simulink model "QPSK_ad9361_Solution"  (R2019a)
settings: Solver=ode23  StartTime=0.0  StopTime=inf  RelTol=1e-3  EnableMultiTasking=on
PreLoadFcn:
  | addpath('./filterwizard');
  | ad9361_preload(bdroot,'rx');
  | sdrqpsktx = qpsktx_init;
  | sdrqpskrx = qpskrx_init;
InitFcn:
  | sdrqpsktx = qpsktx_init;
  | sdrqpskrx = qpskrx_init;
undefined symbols (not defined in the file or in its folder): D, dBc, dBval, DCLeak_Matrix, dfilt, doppler, errordlg, Frame, fuzz_val, GainImb_Matrix, gcbh, IP2_Matrix, IP3_Matrix, magnitude, rcfiltgaincompat
libraries: simrfV2elements x23, dspmlti4 x10, simrfV2util1 x9, simulink x9, dsparch4 x8, fl_lib x7, dspmathops x5, dspobslib x4, simrfV2sources1 x3, simrfV2junction1 x3, commdigbbndpm3 x3, dspstat3 x3
(part 2 of 3)

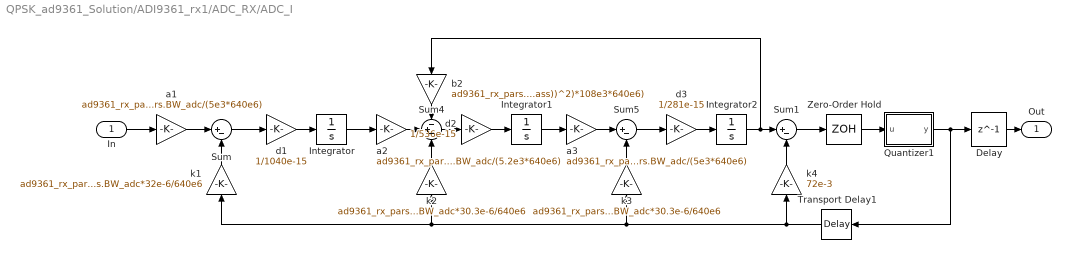
== system QPSK_ad9361_Solution/ADI9361_rx1/ADC_RX/ADC_I ==
  In : Inport
  Delay : Delay  DelayLength=1
  Integrator : Integrator  LimitOutput=on  UpperSaturationLimit=0.9  LowerSaturationLimit=-0.9
  Integrator1 : Integrator  LimitOutput=on  UpperSaturationLimit=0.9  LowerSaturationLimit=-0.9
  Integrator2 : Integrator  LimitOutput=on  UpperSaturationLimit=0.9  LowerSaturationLimit=-0.9
  Quantizer1 : Subsystem
  Sum : Sum  Inputs=|+-
  Sum1 : Sum  Inputs=|+-
  Sum4 : Sum  Inputs=-+-
  Sum5 : Sum  Inputs=|+-
  Transport Delay1 : TransportDelay  DelayTime=ad9361_rx_pars.Tadc/2
  Zero-Order Hold : ZeroOrderHold  SampleTime=ad9361_rx_pars.Tadc
  a1 : Gain  Gain=ad9361_rx_pars.BW_adc/(5e3*640e6)
  a2 : Gain  Gain=ad9361_rx_pars.BW_adc/(5.2e3*640e6)
  a3 : Gain  Gain=ad9361_rx_pars.BW_adc/(5e3*640e6)
  b2 : Gain  Gain=ad9361_rx_pars.BW_adc*1024/(4*((ad9361_rx_pars.BW_adc/(2*ad9361_rx_pars.Fpass))^2)*108e3*640e6)
  d1 : Gain  Gain=1/1040e-15
  d2 : Gain  Gain=1/536e-15
  d3 : Gain  Gain=1/281e-15
  k1 : Gain  Gain=ad9361_rx_pars.BW_adc*32e-6/640e6
  k2 : Gain  Gain=ad9361_rx_pars.BW_adc*30.3e-6/640e6
  k3 : Gain  Gain=ad9361_rx_pars.BW_adc*30.3e-6/640e6
  k4 : Gain  Gain=72e-3
  Out : Outport
  wires:
  k1/1 -> Sum/2
  a1/1 -> Sum/1
  Sum5/1 -> d3/1
  Sum4/1 -> d2/1
  d3/1 -> Integrator2/1
  In/1 -> a1/1
  Integrator2/1 -> Sum1/1, b2/1
  d2/1 -> Integrator1/1
  Integrator1/1 -> a3/1
  d1/1 -> Integrator/1
  Integrator/1 -> a2/1
  Sum/1 -> d1/1
  Zero-Order Hold/1 -> Quantizer1/1(u)
  a2/1 -> Sum4/2
  k2/1 -> Sum4/3
  k3/1 -> Sum5/2
  b2/1 -> Sum4/1
  a3/1 -> Sum5/1
  Sum1/1 -> Zero-Order Hold/1
  k4/1 -> Sum1/2
  Quantizer1/1(y) -> Transport Delay1/1, Delay/1
  Transport Delay1/1 -> k4/1, k1/1, k2/1, k3/1
  Delay/1 -> Out/1

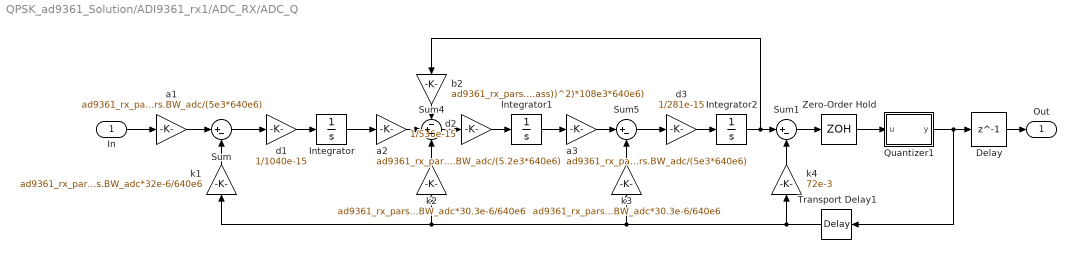
== system QPSK_ad9361_Solution/ADI9361_rx1/ADC_RX/ADC_Q ==
  In : Inport
  Delay : Delay  DelayLength=1
  Integrator : Integrator  LimitOutput=on  UpperSaturationLimit=0.9  LowerSaturationLimit=-0.9
  Integrator1 : Integrator  LimitOutput=on  UpperSaturationLimit=0.9  LowerSaturationLimit=-0.9
  Integrator2 : Integrator  LimitOutput=on  UpperSaturationLimit=0.9  LowerSaturationLimit=-0.9
  Quantizer1 : Subsystem
  Sum : Sum  Inputs=|+-
  Sum1 : Sum  Inputs=|+-
  Sum4 : Sum  Inputs=-+-
  Sum5 : Sum  Inputs=|+-
  Transport Delay1 : TransportDelay  DelayTime=ad9361_rx_pars.Tadc/2
  Zero-Order Hold : ZeroOrderHold  SampleTime=ad9361_rx_pars.Tadc
  a1 : Gain  Gain=ad9361_rx_pars.BW_adc/(5e3*640e6)
  a2 : Gain  Gain=ad9361_rx_pars.BW_adc/(5.2e3*640e6)
  a3 : Gain  Gain=ad9361_rx_pars.BW_adc/(5e3*640e6)
  b2 : Gain  Gain=ad9361_rx_pars.BW_adc*1024/(4*((ad9361_rx_pars.BW_adc/(2*ad9361_rx_pars.Fpass))^2)*108e3*640e6)
  d1 : Gain  Gain=1/1040e-15
  d2 : Gain  Gain=1/536e-15
  d3 : Gain  Gain=1/281e-15
  k1 : Gain  Gain=ad9361_rx_pars.BW_adc*32e-6/640e6
  k2 : Gain  Gain=ad9361_rx_pars.BW_adc*30.3e-6/640e6
  k3 : Gain  Gain=ad9361_rx_pars.BW_adc*30.3e-6/640e6
  k4 : Gain  Gain=72e-3
  Out : Outport
  wires:
  Delay/1 -> Out/1
  Transport Delay1/1 -> k3/1, k2/1, k1/1, k4/1
  Quantizer1/1(y) -> Transport Delay1/1, Delay/1
  k4/1 -> Sum1/2
  Sum1/1 -> Zero-Order Hold/1
  a3/1 -> Sum5/1
  b2/1 -> Sum4/1
  k3/1 -> Sum5/2
  k2/1 -> Sum4/3
  a2/1 -> Sum4/2
  Zero-Order Hold/1 -> Quantizer1/1(u)
  Sum/1 -> d1/1
  Integrator/1 -> a2/1
  d1/1 -> Integrator/1
  Integrator1/1 -> a3/1
  d2/1 -> Integrator1/1
  Integrator2/1 -> b2/1, Sum1/1
  In/1 -> a1/1
  d3/1 -> Integrator2/1
  Sum4/1 -> d2/1
  Sum5/1 -> d3/1
  a1/1 -> Sum/1
  k1/1 -> Sum/2

== system QPSK_ad9361_Solution/ADI9361_rx1/Average Power Meter/Peak Detector ==
  In : Inport
  HTh_i : Constant  Value=Hthreshold_i  SampleTime=ad9361_rx_pars.Tpow*Ncycles
  HTh_o : Constant  Value=Hthreshold_o  SampleTime=ad9361_rx_pars.Tpow*Ncycles
  HighThreshold : RelationalOperator  OutDataTypeStr=boolean  RndMeth=Nearest
  HighThreshold1 : RelationalOperator  Operator=<=  OutDataTypeStr=boolean  RndMeth=Nearest
  LTh_i : Constant  Value=Lthreshold_i  SampleTime=ad9361_rx_pars.Tpow*Ncycles
  LTh_o : Constant  Value=Lthreshold_o  SampleTime=ad9361_rx_pars.Tpow*Ncycles
  LowThreshold : RelationalOperator  OutDataTypeStr=boolean  RndMeth=Nearest
  LowThreshold1 : RelationalOperator  Operator=<=  OutDataTypeStr=boolean  RndMeth=Nearest
  Outer_HTh : Outport
  Inner_HTh : Outport  Port=2
  Inner_LTh : Outport  Port=3
  Outer_LTh : Outport  Port=4
  wires:
  LowThreshold/1 -> Inner_HTh/1
  HighThreshold/1 -> Outer_HTh/1
  HTh_i/1 -> LowThreshold/2
  HTh_o/1 -> HighThreshold/2
  LTh_o/1 -> LowThreshold1/2
  In/1 -> HighThreshold/1, LowThreshold1/1, HighThreshold1/1, LowThreshold/1
  LTh_i/1 -> HighThreshold1/2
  HighThreshold1/1 -> Inner_LTh/1
  LowThreshold1/1 -> Outer_LTh/1

== system QPSK_ad9361_Solution/ADI9361_rx1/Average Power Meter/RMS ==
  In : Inport
  CountNCycles : Buffer  N=Ncycles
  Frame Conversion : FrameConversion  OutFrame=Sample-based
  Gain2 : Gain  Gain=1/Ncycles
  Root : Sqrt  SaturateOnIntegerOverflow=on
  Squared : Math  Operator=magnitude^2  SaturateOnIntegerOverflow=on
  Sum : Sum  Inputs=+
  Out : Outport
  wires:
  Sum/1 -> Gain2/1
  Frame Conversion/1 -> Out/1
  CountNCycles/1 -> Squared/1
  Squared/1 -> Sum/1
  Root/1 -> Frame Conversion/1
  Gain2/1 -> Root/1
  In/1 -> CountNCycles/1

== system QPSK_ad9361_Solution/ADI9361_rx1/Average Power Meter/dB Conversion ==
  in : Inport
  Constant : Constant  Value=fuzz_val  OutDataTypeStr=Inherit: Inherit via back propagation  SampleTime=ad9361_rx_pars.Tpow*Ncycles
  Constant1 : Constant  Value=dBval  OutDataTypeStr=Inherit: Inherit via back propagation  SampleTime=ad9361_rx_pars.Tpow*Ncycles
  Err if non-flt : dspsigattribs/Check Signal Attributes  SigAttribCheckMethod=Does not match attributes exactly  Complexity=Ignore  Frame=Ignore  DimsCheckMethod=Ignore  Dimensions=1-D  DatatypeCheckMethod=Is...  DatatypeGeneral=Floating-point  DtypeFloatSpecific=Any floating-point  DtypeFixedSpecific=Any fixed-point  DtypeIntSpecific=Any integer  SampleMode=Ignore
      settings: SourceProductName=DSP System Toolbox  SourceProductBaseCode=DS
  Error if Cplx : dspsigattribs/Check Signal Attributes  SigAttribCheckMethod=Matches attributes exactly  Complexity=Complex  Frame=Ignore  DimsCheckMethod=Ignore  Dimensions=1-D  DatatypeCheckMethod=Ignore  DatatypeGeneral=Boolean  DtypeFloatSpecific=Any floating-point  DtypeFixedSpecific=Any fixed-point  DtypeIntSpecific=Any integer  SampleMode=Ignore
      settings: SourceProductName=DSP System Toolbox  SourceProductBaseCode=DS
  Gain : Gain  Gain=10  SaturateOnIntegerOverflow=on  OutDataTypeStr=Inherit: Same as input  ParamDataTypeStr=Inherit: Same as input
  Magsq : Math  Operator=magnitude^2  SaturateOnIntegerOverflow=on
  Scale by R : Gain  Gain=1./R  SaturateOnIntegerOverflow=on  OutDataTypeStr=Inherit: Same as input  ParamDataTypeStr=Inherit: Same as input
  Sum1 : Sum  SaturateOnIntegerOverflow=on  InputSameDT=on  OutDataTypeStr=Inherit: Same as first input
  Sum2 : Sum  SaturateOnIntegerOverflow=on  InputSameDT=on  OutDataTypeStr=Inherit: Same as first input
  log10 : Math  Operator=log10  SaturateOnIntegerOverflow=on
  out : Outport  InitialOutput=0
  wires:
  log10/1 -> Gain/1
  Magsq/1 -> Scale by R/1
  Scale by R/1 -> log10/1
  Err if non-flt/1 -> Error if Cplx/1
  in/1 -> Err if non-flt/1
  Error if Cplx/1 -> Sum1/1
  Sum1/1 -> Magsq/1
  Constant/1 -> Sum1/2
  Gain/1 -> Sum2/1
  Sum2/1 -> out/1
  Constant1/1 -> Sum2/2

== system QPSK_ad9361_Solution/ADI9361_rx1/DDC_Filters_RX/Hm1 ==
  note: 1) Only subsystems can be added as variant choices at this level
      | 2) Blocks cannot be connected at this level as connectivity is
      | automatically determined at simulation, based on the active variant
  In : Inport
  Hm1 : Subsystem  VariantControl=(default)
  NoFilter : Subsystem  VariantControl=ad9361_rx_hm1Filt==0
  Out : Outport

== system QPSK_ad9361_Solution/ADI9361_rx1/DDC_Filters_RX/Hm2 ==
  note: 1) Only subsystems can be added as variant choices at this level
      | 2) Blocks cannot be connected at this level as connectivity is
      | automatically determined at simulation, based on the active variant
  In : Inport
  Hm2 : Subsystem  VariantControl=(default)
  NoFilter : Subsystem  VariantControl=ad9361_rx_hm2Filt==0
  Out : Outport

== system QPSK_ad9361_Solution/ADI9361_rx1/DDC_Filters_RX/Hm3 ==
  note: 1) Only subsystems can be added as variant choices at this level
      | 2) Blocks cannot be connected at this level as connectivity is
      | automatically determined at simulation, based on the active variant
  In : Inport
  Hm3 : Subsystem  VariantControl=(default)
  NoFilter : Subsystem  VariantControl=ad9361_rx_hm3Filt==0
  Out : Outport

== system QPSK_ad9361_Solution/ADI9361_rx1/DDC_Filters_RX/Hm4 ==
  note: 1) Only subsystems can be added as variant choices at this level
      | 2) Blocks cannot be connected at this level as connectivity is
      | automatically determined at simulation, based on the active variant
  In1 : Inport
  Hm4 : Subsystem  VariantControl=(default)
  NoFilter : Subsystem  VariantControl=ad9361_rx_hm4Filt==0
  Out1 : Outport

== system QPSK_ad9361_Solution/ADI9361_rx1/LPF_RX/dB2lin ==
  In : Inport
  1/20 : Gain  Gain=1/20
  exp : Math  Operator=10^u  SaturateOnIntegerOverflow=on
  Out : Outport
  wires:
  exp/1 -> Out/1
  In/1 -> 1/20/1
  1/20/1 -> exp/1

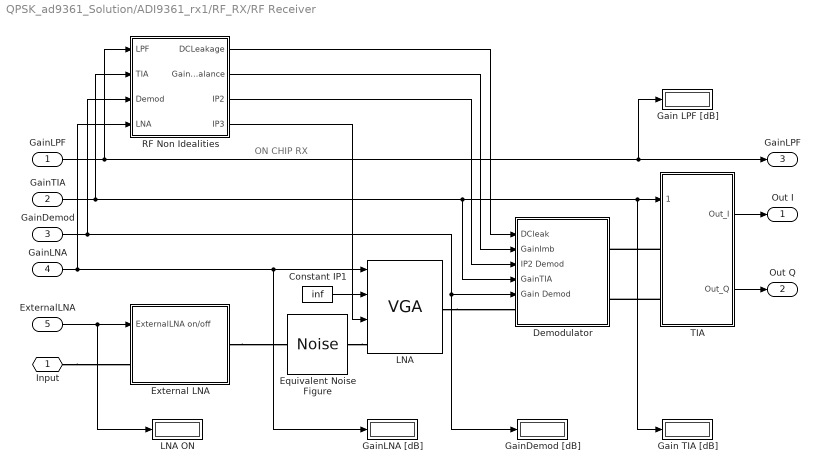
== system QPSK_ad9361_Solution/ADI9361_rx1/RF_RX/RF Receiver ==
  note: ON CHIP RX
  GainLPF : Inport
  GainTIA : Inport  Port=2
  GainDemod : Inport  Port=3
  GainLNA : Inport  Port=4
  ExternalLNA : Inport  Port=5
  Constant IP1 : Constant  Value=inf
  Demodulator : Subsystem
  Equivalent Noise Figure : simrfV2sources1/Noise  SimulinkInputSignalType=Ideal voltage  NoiseType=White  NoisePSD=4*1.381e-23*290*50*10^(NF/10)  CarrierFreq=fc_RF Hz  InternalGrounding=off
      settings: SourceProductName=RF Blockset  SourceProductBaseCode=RB
  External LNA : Subsystem
  Gain LPF [dB] : Display
  Gain TIA [dB] : Display
  GainDemod [dB] : Display
  GainLNA [dB] : Display
  LNA : simrfV2elements/VGA  classname=vga  Zin=Rin  Zout=50  IO=Input  InternalGrounding=on
      settings: SourceProductName=RF Blockset  SourceProductBaseCode=RB
  LNA ON : Display
  RF Non Idealities : Subsystem
  TIA : Subsystem
  Input : PMIOPort  Side=Left
  Out I : Outport
  Out Q : Outport  Port=2
  "GainLPF " : Outport  Port=3
  wires:
  GainTIA/1 -> RF Non Idealities/2(TIA), Gain TIA [dB]/1, TIA/1(Gain TIA), Demodulator/4(GainTIA)
  TIA/1(Out_I) -> Out I/1
  TIA/2(Out_Q) -> Out Q/1
  GainDemod/1 -> RF Non Idealities/3(Demod), Demodulator/5(Gain Demod), GainDemod [dB]/1
  GainLNA/1 -> LNA/1, GainLNA [dB]/1, RF Non Idealities/4(LNA)
  GainLPF/1 -> "GainLPF "/1, Gain LPF [dB]/1, RF Non Idealities/1(LPF)
  RF Non Idealities/1(DCLeakage) -> Demodulator/1(DCleak)
  RF Non Idealities/3(IP2) -> Demodulator/3(IP2 Demod)
  RF Non Idealities/4(IP3) -> LNA/3
  Constant IP1/1 -> LNA/2
  ExternalLNA/1 -> LNA ON/1, External LNA/1(ExternalLNA on/off)
  RF Non Idealities/2(GainImbalance) -> Demodulator/2(GainImb)
  connections:
  LNA/RConn1 -- Demodulator/LConn1
  TIA/LConn1 -- Demodulator/RConn1
  TIA/LConn2 -- Demodulator/RConn2
  Equivalent Noise Figure/LConn1 -- LNA/LConn1
  Input/RConn1 -- External LNA/LConn1
  External LNA/RConn1 -- Equivalent Noise Figure/RConn1

== system QPSK_ad9361_Solution/ADI9361_rx1/Subsystem6/Subsystem1 ==
  Data Type Conversion : DataTypeConversion  OutDataTypeStr=boolean
  Pulse Generator2 : DiscretePulseGenerator  SampleTime=Trf
  START : Outport
  wires:
  Pulse Generator2/1 -> Data Type Conversion/1
  Data Type Conversion/1 -> START/1

== system QPSK_ad9361_Solution/ADI9361_rx1/Subsystem6/Subsystem2 ==
  s : Inport
  w : Inport  Port=2
  Data Type Conversion : DataTypeConversion  OutDataTypeStr=boolean
  Subtract1 : Sum  Inputs=-+  OutDataTypeStr=int8
  os : Outport
  ow : Outport  Port=2
  wires:
  s/1 -> Subtract1/2, os/1
  Data Type Conversion/1 -> ow/1
  Subtract1/1 -> Data Type Conversion/1
  w/1 -> Subtract1/1

== system QPSK_ad9361_Solution/ADI9361_rx1/Subsystem6/Subsystem3 ==
  w : Inport
  s : Inport  Port=2
  Data Type Conversion : DataTypeConversion  OutDataTypeStr=boolean
  Subtract1 : Sum  Inputs=-+  OutDataTypeStr=int8
  ow : Outport
  os : Outport  Port=2
  wires:
  w/1 -> Subtract1/1
  Subtract1/1 -> Data Type Conversion/1
  Data Type Conversion/1 -> ow/1
  s/1 -> Subtract1/2, os/1

== system QPSK_ad9361_Solution/ADI9361_rx1/Subsystem6/Wblk4 ==
  Win : Inport
  Sin : Inport  Port=2
  Combinatorial Logic : CombinatorialLogic  TruthTable=[0; 0; 1; 0]
  Mux : Mux  Inputs=2
  Wout : Outport
  wires:
  Mux/1 -> Combinatorial Logic/1
  Combinatorial Logic/1 -> Wout/1  "wout"
  Win/1 -> Mux/1
  Sin/1 -> Mux/2

== system QPSK_ad9361_Solution/ADI9361_rx1/Subsystem6/Wblk4a ==
  Win : Inport
  Sin : Inport  Port=2
  Combinatorial Logic : CombinatorialLogic  TruthTable=[0; 0; 1; 0]
  Mux : Mux  Inputs=2
  Wout : Outport
  wires:
  Mux/1 -> Combinatorial Logic/1
  Combinatorial Logic/1 -> Wout/1  "wout"
  Win/1 -> Mux/1
  Sin/1 -> Mux/2

== system QPSK_ad9361_Solution/ADI9361_rx1/Subsystem6/Wblk5 ==
  Win : Inport
  Sin : Inport  Port=2
  Combinatorial Logic : CombinatorialLogic  TruthTable=[0; 0; 1; 0]
  Mux : Mux  Inputs=2
  Wout : Outport
  wires:
  Mux/1 -> Combinatorial Logic/1
  Combinatorial Logic/1 -> Wout/1  "wout"
  Win/1 -> Mux/1
  Sin/1 -> Mux/2

== system QPSK_ad9361_Solution/ADI9361_rx1/Subsystem6/Wblk6 ==
  Win : Inport
  Sin : Inport  Port=2
  Combinatorial Logic : CombinatorialLogic  TruthTable=[0; 0; 1; 0]
  Mux : Mux  Inputs=2
  Wout : Outport
  wires:
  Mux/1 -> Combinatorial Logic/1
  Combinatorial Logic/1 -> Wout/1  "wout"
  Win/1 -> Mux/1
  Sin/1 -> Mux/2

== system QPSK_ad9361_Solution/ADI9361_rx1/Subsystem6/Wblk7 ==
  Win : Inport
  Sin : Inport  Port=2
  Combinatorial Logic : CombinatorialLogic  TruthTable=[0; 0; 1; 0]
  Mux : Mux  Inputs=2
  Wout : Outport
  wires:
  Mux/1 -> Combinatorial Logic/1
  Combinatorial Logic/1 -> Wout/1  "wout"
  Win/1 -> Mux/1
  Sin/1 -> Mux/2

== system QPSK_ad9361_Solution/ADI9361_tx1/DUC_Filters_TX/Hm1 ==
  note: 1) Only subsystems can be added as variant choices at this level
      | 2) Blocks cannot be connected at this level as connectivity is
      | automatically determined at simulation, based on the active variant
  In : Inport
  Hm1 : Subsystem  VariantControl=(default)
  NoFilter : Subsystem  VariantControl=ad9361_tx_hm1Filt==0
  Out : Outport

== system QPSK_ad9361_Solution/ADI9361_tx1/DUC_Filters_TX/Hm2 ==
  note: 1) Only subsystems can be added as variant choices at this level
      | 2) Blocks cannot be connected at this level as connectivity is
      | automatically determined at simulation, based on the active variant
  In : Inport
  Hm2 : Subsystem  VariantControl=(default)
  NoFilter : Subsystem  VariantControl=ad9361_tx_hm2Filt==0
  Out : Outport

== system QPSK_ad9361_Solution/ADI9361_tx1/DUC_Filters_TX/Hm3 ==
  note: 1) Only subsystems can be added as variant choices at this level
      | 2) Blocks cannot be connected at this level as connectivity is
      | automatically determined at simulation, based on the active variant
  In : Inport
  Hm3 : Subsystem  VariantControl=(default)
  NoFilter : Subsystem  VariantControl=ad9361_tx_hm3Filt==0
  Out : Outport

== system QPSK_ad9361_Solution/ADI9361_tx1/DUC_Filters_TX/Hm4 ==
  note: 1) Only subsystems can be added as variant choices at this level
      | 2) Blocks cannot be connected at this level as connectivity is
      | automatically determined at simulation, based on the active variant
  In1 : Inport
  Hm4 : Subsystem  VariantControl=(default)
  NoFilter : Subsystem  VariantControl=ad9361_tx_hm4Filt==0
  Out1 : Outport

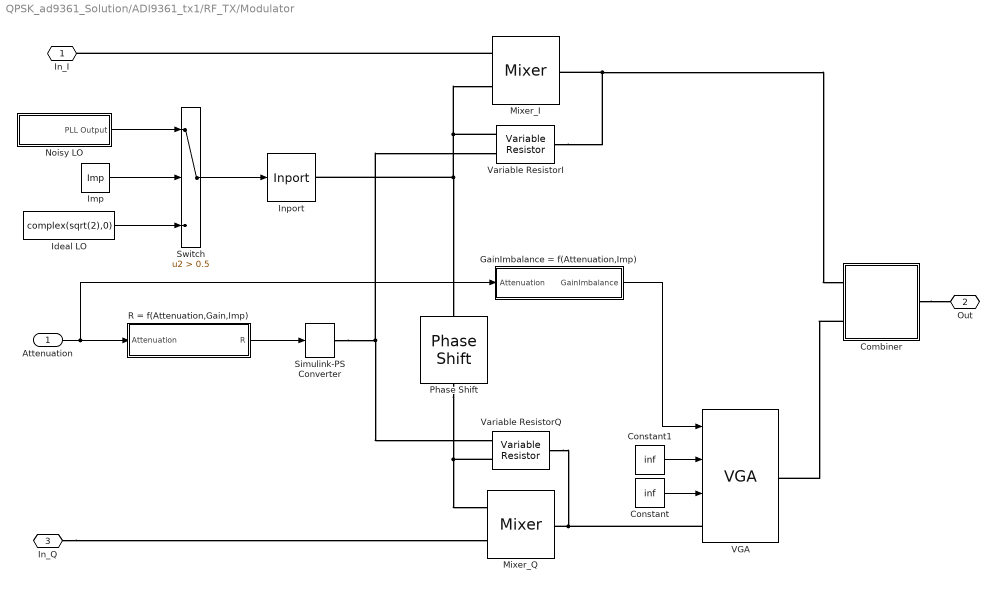
== system QPSK_ad9361_Solution/ADI9361_tx1/RF_TX/Modulator ==
  Attenuation : Inport
  Combiner : Subsystem
  Constant : Constant  Value=inf
  Constant1 : Constant  Value=inf
  GainImbalance = f(Attenuation,Imp) : Subsystem
  Ideal LO : Constant  Value=complex(sqrt(2),0)  SampleTime=Tstep
  Imp : Constant  Value=Imp  SampleTime=Tstep
  Inport : simrfV2util1/Inport  SimulinkInputSignalType=Ideal voltage  CarrierFreq=RF Hz  ZS=0  InternalGrounding=on
      settings: SourceProductName=RF Blockset  SourceProductBaseCode=RB
  Mixer_I : simrfV2elements/Mixer  classname=mixer  Source_linear_gain=Available power gain  linear_gain=0 dB  Zin=50  Zout=50  ZLO=inf  Source_Poly=Even and odd order  Poly_Coeffs=[0 1]  IPType=Output  IP2=Inf dBm  IP3=Inf dBm  P1dB=Inf dBm  Psat=Inf dBm  Gcomp=Inf dBm  NF=0  InternalGrounding=on
      settings: SourceProductName=RF Blockset  SourceProductBaseCode=RB
  Mixer_Q : simrfV2elements/Mixer  classname=mixer  Source_linear_gain=Available power gain  linear_gain=0 dB  Zin=50  Zout=50  ZLO=inf  Source_Poly=Even and odd order  Poly_Coeffs=[0 1]  IPType=Output  IP2=Inf dBm  IP3=Inf dBm  P1dB=Inf dBm  Psat=Inf dBm  Gcomp=Inf dBm  NF=0  InternalGrounding=on
      settings: SourceProductName=RF Blockset  SourceProductBaseCode=RB
  Noisy LO : Subsystem  mask{Level_dB=PN-6, Freq=freqPN, Fs=1/Tstep, Npts=1024*16, seed=951357}
      mask prompts: Level_dB "Noise Level Vector in dBc/Hz"; Freq "Frequency Vector in Hz"; Fs "Sampling Rate in Hz"; Npts "FIR Filter Kernel Length"; seed "Noise Gen Seed"
  Phase Shift : simrfV2elements/Phase Shift  PhaseShift=90 deg  InternalGrounding=on
      settings: SourceProductName=RF Blockset  SourceProductBaseCode=RB
  R = f(Attenuation,Gain,Imp) : Subsystem
  Simulink-PS Converter : nesl_utility/Simulink-PS Converter  PhysicalDomain=network_engine_domain  SubClassName=ps_input  LeftPortType=input  RightPortType=output  PseudoPeriodic=off  Frequencies=[]  NoiseDistribution=none  NoiseParameters=[]  Unit=1  AffineConversion=off  InputFiltering=off  SimscapeFilterOrder=1  InputFilterTimeConstant=0.001  UdotUserProvided=1
  Switch : Switch  Criteria=u2 > Threshold  Threshold=0.5
  VGA : simrfV2elements/VGA  classname=vga  Zin=50  Zout=50  IO=Input  InternalGrounding=on
      settings: SourceProductName=RF Blockset  SourceProductBaseCode=RB
  Variable ResistorI : fl_lib/Electrical/Electrical Elements/Variable Resistor  Rmin=0 Ohm  i_specify=off  i_priority=None  i=0 A  v_specify=off  v_priority=None  v=0 V
  Variable ResistorQ : fl_lib/Electrical/Electrical Elements/Variable Resistor  Rmin=0 Ohm  i_specify=off  i_priority=None  i=0 A  v_specify=off  v_priority=None  v=0 V
  In_I : PMIOPort  Side=Left
  Out : PMIOPort  Port=2  Side=Right
  In_Q : PMIOPort  Port=3  Side=Left
  wires:
  R = f(Attenuation,Gain,Imp)/1(R) -> Simulink-PS Converter/1
  Attenuation/1 -> R = f(Attenuation,Gain,Imp)/1(Attenuation), GainImbalance = f(Attenuation,Imp)/1(Attenuation)
  Switch/1 -> Inport/1
  Imp/1 -> Switch/2
  Noisy LO/1(PLL Output) -> Switch/1
  Ideal LO/1 -> Switch/3
  GainImbalance = f(Attenuation,Imp)/1(GainImbalance) -> VGA/1
  Constant1/1 -> VGA/2
  Constant/1 -> VGA/3
  connections:
  Phase Shift/RConn1 -- Variable ResistorQ/LConn2 -- Mixer_Q/LConn2
  Mixer_I/LConn1 -- In_I/RConn1
  Inport/RConn1 -- Phase Shift/LConn1 -- Variable ResistorI/LConn2 -- Mixer_I/LConn2
  In_Q/RConn1 -- Mixer_Q/LConn1
  Simulink-PS Converter/RConn1 -- Variable ResistorQ/LConn1 -- Variable ResistorI/LConn1
  Variable ResistorQ/RConn1 -- VGA/LConn1 -- Mixer_Q/RConn1
  Variable ResistorI/RConn1 -- Mixer_I/RConn1 -- Combiner/LConn1
  Combiner/RConn1 -- Out/RConn1
  Combiner/LConn2 -- VGA/RConn1

== system QPSK_ad9361_Solution/ADI9361_tx1/RF_TX/PA ==
  " Attenuation" : Inport
  Constant : Constant  Value=Gain
  Constant1 : Constant  Value=inf
  Equivalent Noise Figure : simrfV2sources1/Noise  SimulinkInputSignalType=Ideal voltage  NoiseType=White  NoisePSD=4*1.381e-23*290*50*10^(NF/10)  CarrierFreq=fc_RF Hz  InternalGrounding=off
      settings: SourceProductName=RF Blockset  SourceProductBaseCode=RB
  OIP3 = f(Attenuation,OIP3v,Imp) : Subsystem
  VGA : simrfV2elements/VGA  classname=vga  Zin=50  Zout=50  IO=Output  InternalGrounding=on
      settings: SourceProductName=RF Blockset  SourceProductBaseCode=RB
  In : PMIOPort  Side=Left
  Out : PMIOPort  Port=2  Side=Right
  wires:
  Constant/1 -> VGA/1
  " Attenuation"/1 -> OIP3 = f(Attenuation,OIP3v,Imp)/1(Attenuation)
  OIP3 = f(Attenuation,OIP3v,Imp)/1(OIP3) -> VGA/3
  Constant1/1 -> VGA/2
  connections:
  In/RConn1 -- VGA/LConn1
  Equivalent Noise Figure/RConn1 -- VGA/RConn1
  Equivalent Noise Figure/LConn1 -- Out/RConn1

== system QPSK_ad9361_Solution/QPSK Receiver/Coarse Frequency Compensation1/Find Frequency Offset ==
  note: Algorithm:
      | 1.  Introduce nonlinearity to create tone at M*Foffset, where M is modulation order
      | 2.  Find index of tone within FFT vector
      | 3.  Compute frequency offset
  In : Inport
  Alphabet size : Constant  Value=M  OutDataTypeStr=Inherit: Inherit via back propagation
  Complex Power : commblksprivate/Complex Power
      settings: SourceProductName=Communications Toolbox  SourceProductBaseCode=CM
  Find Frequency Offset : MATLAB Function  TreatAsAtomicUnit=on
  Periodogram : dspspect3/Periodogram  measurement=Power spectral density  wintype=Hamming  Rs=50  beta=5  winsamp=Symmetric  FFTImplementation=Auto  inheritFFT=off  fftsize=2048  navg=16  inheritTs=on  Ts=1
      settings: SourceProductName=DSP System Toolbox  SourceProductBaseCode=DS
  Probe : Probe  ProbeComplexSignal=off
  Frq : Outport
  wires:
  Periodogram/1 -> Find Frequency Offset/3(FFTSig)
  Alphabet size/1 -> Complex Power/2
  In/1 -> Complex Power/1
  Probe/1 -> Find Frequency Offset/1(N)
  Probe/2 -> Find Frequency Offset/2(Tf)
  Find Frequency Offset/1(FreqOffset) -> Frq/1
  Complex Power/1 -> Probe/1, Periodogram/1

== system QPSK_ad9361_Solution/QPSK Receiver/Data Decoding1/Barker Code Symbol Generation  ==
  note: Regenerate a QPSK-modulated unipolar Barker code sequence
      | to be compared with the received data
  Constant Barker Code : Constant  Value=|  VectorParams1D=off
      | [+1 +1 +1 +1 +1 -1 -1 +1 +1 -1 +1 -1 +1
      | ].' > 0
      settings: SamplingMode=Frame based
  Data Type Conversion : DataTypeConversion  OutDataTypeStr=double
  QPSK Modulator Baseband : commdigbbndpm3/QPSK Modulator Baseband  InType=Bit  Enc=Gray  Ph=pi/4  outDtype=double  outWordLen=16  outUDDataType=sfix(16)  outFracLenMode=Best precision  outFracLen=15  outDataTypeStr=double  outLastDataTypeStr=double
      settings: SourceProductName=Communications Toolbox
  Repeat : dspsigops/Repeat  N=2  InputProcessing=Columns as channels (frame based)  RateOptions=Enforce single-rate processing  ic=0  mode=Unused parameter value
      settings: SourceProductName=DSP System Toolbox
  Out : Outport
  wires:
  Constant Barker Code/1 -> Data Type Conversion/1
  Repeat/1 -> QPSK Modulator Baseband/1
  QPSK Modulator Baseband/1 -> Out/1
  Data Type Conversion/1 -> Repeat/1

== system QPSK_ad9361_Solution/QPSK Receiver/Data Decoding1/Compute Delay ==
  note: Correlation with the modulated symbols
  Barker Reference : Inport
  Data : Inport  Port=2
  Abs : Abs
  Constant1 : Constant  VectorParams1D=off  OutDataTypeStr=Inherit: Inherit via back propagation  FramePeriod=2
  Correlation : dspstat3/Correlation  domain=Time  roundingMode=Floor  overflowMode=off  accumDataTypeStr=Inherit: Same as product output  accumLastDataTypeStr=Inherit: Same as product output  outputDataTypeStr=Inherit: Same as accumulator  outputMin=[]  outputMax=[]  outputLastDataTypeStr=Inherit: Same as accumulator
      settings: SourceProductName=DSP System Toolbox  SourceProductBaseCode=DS
  Math Function : Math  Operator=mod  SaturateOnIntegerOverflow=on
  Maximum : dspstat3/Maximum  operation=maximum  fcn=Index  indexBase=One  operateOver=Each column  Dimension=1  InputProcessing=Columns as channels (frame based)  reset=None  roiEnable=off  roiType=Rectangles  roiPortion=Entire ROI  roiOutput=Individual statistics for each ROI  roiFlag=off  roundingMode=Floor  overflowMode=off  accumDataTypeStr=Inherit: Same as product output  accumLastDataTypeStr=Inherit: Same as product output
  Probe : Probe  ProbeSampleTime=off  ProbeComplexSignal=off
  Sum : Sum  Inputs=|-+  SaturateOnIntegerOverflow=on  InputSameDT=on  OutDataTypeStr=Inherit: Same as first input
  Sum1 : Sum  Inputs=|+-  SaturateOnIntegerOverflow=on  InputSameDT=on  OutDataTypeStr=Inherit: Same as first input
  Delay : Outport
  wires:
  Abs/1 -> Maximum/1
  Constant1/1 -> Sum1/2
  Sum1/1 -> Math Function/2
  Math Function/1 -> Delay/1
  Sum/1 -> Math Function/1
  Probe/1 -> Sum1/1, Sum/2
  Correlation/1 -> Abs/1
  Maximum/1 -> Sum/1
  Barker Reference/1 -> Correlation/1
  Data/1 -> Correlation/2, Probe/1

== system QPSK_ad9361_Solution/QPSK Receiver/Data Decoding1/Descrambling ==
  In : Inport
  Descrambler : commsequence2/Descrambler  M=2  poly=[1 1 1 0 1]  iniStaSource=Dialog Parameter  ini_sta=[0 0 0 0]  resetViaPort=off
      settings: SourceProductName=Communications Toolbox  SourceProductBaseCode=CM
  Selector : Selector  IndexOptions=Index vector (dialog)  Indices=[sdrqpskrx.BarkerLength*log2(sdrqpskrx.M)+1:sdrqpskrx.FrameSize*log2(sdrqpskrx.M)]  OutputSizes=1
  Selector1 : Selector  IndexOptions=Index vector (dialog)  Indices=[1:sdrqpskrx.MsgLength]  OutputSizes=1
  Out : Outport
  wires:
  Descrambler/1 -> Selector1/1
  Selector1/1 -> Out/1
  In/1 -> Selector/1
  Selector/1 -> Descrambler/1

== system QPSK_ad9361_Solution/QPSK Receiver/Data Decoding1/Phase Ambiguity Correction & Demodulation ==
  note: Phase Ambiguity Resolution
      | and Demodulation
  Phase : Inport
  Data : Inport  Port=2
  Complex Phase Shift : commutil2/Complex Phase Shift
      settings: SourceProductName=Communications Toolbox  SourceProductBaseCode=CM
  Constellation RX : ConstellationDiagram
  Gain : Gain  Gain=-1
  QPSK Demodulator Baseband : commdigbbndpm3/QPSK Demodulator Baseband  OutType=Bit  DecType=Hard decision  VarSource=Dialog  Variance=1  Dec=Gray  Ph=pi/4  outDtype1=Inherit via internal rule  outDtype2=Inherit via internal rule  derotateFactorWordLen=16  derotateFactorDataTypeStr=Inherit: Same word length as input  derotateFactorLastDataTypeStr=Inherit: Same word length as input
      settings: SourceProductName=Communications Toolbox
  Out : Outport
  wires:
  Phase/1 -> Gain/1
  Data/1 -> Complex Phase Shift/1
  Complex Phase Shift/1 -> Constellation RX/1, QPSK Demodulator Baseband/1
  QPSK Demodulator Baseband/1 -> Out/1
  Gain/1 -> Complex Phase Shift/2

== system QPSK_ad9361_Solution/QPSK Receiver/Data Decoding1/Phase Offset Estimator ==
  note: 1. The original signal is expressed as y(t) = x(t)e^{j\phi}+n(t), t = 1, 2, ..., N
      | 2. y_1(t) = x{*}(t)y(t) = e^{j\phi} + x{*}(t)n(t)
      | The goal is to estimate the value \phi from the observation y_1(t), t = 1, 2, ...N
      | i.e., estimate the value B = e^{j\phi}, and \phi = angle(B)
      | 3. Suppose n(t) yields to a i.i.d. complex AWGN distribution N(0,\sigma^2).
      | Then a non-biased estimator could be
      | B_{est} = 1/N*sum(y_1(1:N)), and \phi_{est} = angle(B_{est})
      | and the variance of B_{est} is \sigma^2/N
  BarkerRef : Inport
  Data : Inport  Port=2
  Complex to Magnitude-Angle : ComplexToMagnitudeAngle  Output=Angle
  Math Function : Math  Operator=conj  SaturateOnIntegerOverflow=on
  Mean : dspstat3/Mean  run=off  reset_popup=None  InputProcessing=Columns as channels (frame based)  directionMode=Each column  dimension=1  roiEnable=off  roiType=Rectangles  roiPortion=Entire ROI  roiOutput=Individual statistics for each ROI  roiFlag=off  outputDataTypeStr=Inherit: Same as accumulator  outputLastDataTypeStr=Inherit: Same as accumulator  outputMin=[]  outputMax=[]  roundingMode=Floor  overflowMode=off
  Phase Offset Detection : MATLAB Function  TreatAsAtomicUnit=on
  Product : Product  RndMeth=Zero
  Selector : Selector  IndexOptions=Index vector (dialog)  Indices=[1:sdrqpskrx.BarkerLength]  OutputSizes=1
  Phase : Outport
  wires:
  Data/1 -> Selector/1
  BarkerRef/1 -> Math Function/1  "x(t)"
  Selector/1 -> Product/2  "y(t)"
  Math Function/1 -> Product/1  "x*(t)"
  Product/1 -> Mean/1  "y_1(t)"
  Mean/1 -> Complex to Magnitude-Angle/1
  Complex to Magnitude-Angle/1 -> Phase Offset Detection/1(In)
  Phase Offset Detection/1(Out) -> Phase/1

== system QPSK_ad9361_Solution/QPSK Receiver/Fine Frequency Compensation1/DDS ==
  note: The digital filter acts as a pure integrator
  In : Inport
  Digital Filter : dspobslib/Digital Filter  TypePopup=IIR (poles & zeros)  IIRFiltStruct=Direct form II transposed  AllPoleFiltStruct=Direct form  FIRFiltStruct=Direct form  CoeffSource=Specify via dialog  NumCoeffs=[0 1]  DenCoeffs=[1 -1]  BiQuadCoeffs=[1 0.3 0.4 1 0.1 0.2]  LatticeCoeffs=[0.2 0.4]  denIgnore=on  FiltPerSampPopup=One filter per frame  IC=0  ICnum=0  ICden=0  roundingMode=Floor  overflowMode=off  ScaleValues=1  scaleValueFracLength=14  stageInFracLength=15  stageOutFracLength=15  FilterSource=Specify via dialog  dfiltObjectName=dfilt.dffir([1 2 1])  InputProcessing=Columns as channels (frame based)
      settings: SourceProductName=DSP System Toolbox  SourceProductBaseCode=DS
  Gain : Gain  Gain=-1*sdrqpskrx.FineFreqCompensateGain
  Phase : Outport
  wires:
  Digital Filter/1 -> Gain/1
  In/1 -> Digital Filter/1
  Gain/1 -> Phase/1

== system QPSK_ad9361_Solution/QPSK Receiver/Fine Frequency Compensation1/Loop Filter ==
  note: Proportional-plus-Integrator Loop Filter,
      | Infinite DC Response to guarantee convergence
  e : Inport
  Digital Filter : dspobslib/Digital Filter  TypePopup=IIR (poles & zeros)  IIRFiltStruct=Direct form II transposed  AllPoleFiltStruct=Direct form  FIRFiltStruct=Direct form  CoeffSource=Specify via dialog  NumCoeffs=[1 0]  DenCoeffs=[1 -1]  BiQuadCoeffs=[1 0.3 0.4 1 0.1 0.2]  LatticeCoeffs=[0.2 0.4]  denIgnore=on  FiltPerSampPopup=One filter per frame  IC=0  ICnum=0  ICden=0  roundingMode=Floor  overflowMode=off  ScaleValues=1  scaleValueFracLength=14  stageInFracLength=15  stageOutFracLength=15  FilterSource=Specify via dialog  dfiltObjectName=dfilt.dffir([1 2 1])  InputProcessing=Columns as channels (frame based)
      settings: SourceProductName=DSP System Toolbox  SourceProductBaseCode=DS
  K1 : Gain  Gain=K1
  K2 : Gain  Gain=K2
  Sum2 : Sum  SaturateOnIntegerOverflow=on  InputSameDT=on  OutDataTypeStr=Inherit: Same as first input
  v : Outport
  wires:
  K2/1 -> Digital Filter/1
  Digital Filter/1 -> Sum2/2
  Sum2/1 -> v/1
  e/1 -> K2/1, K1/1
  K1/1 -> Sum2/1

== system QPSK_ad9361_Solution/QPSK Receiver/Timing Recovery1/Modified Buffer ==
  Data : Inport
  Clk : Inport  Port=2
  Logical Operator : Logic  AllPortsSameDT=off  OutDataTypeStr=boolean
  Modified Buffer : Subsystem
  DataOut : Outport
  DataValid : Outport  Port=2
  wires:
  Data/1 -> Modified Buffer/1(In1)
  Clk/1 -> Modified Buffer/Enable, Logical Operator/2
  Modified Buffer/1(DataOut) -> DataOut/1
  Modified Buffer/2(DataValid) -> Logical Operator/1
  Logical Operator/1 -> DataValid/1

== system QPSK_ad9361_Solution/QPSK Receiver/Timing Recovery1/Timing Recovery PLL ==
  note: Sample-based processing is adopted because
      | 1. Strobe signal is required to generate for EVERY sample for processing and output
      | sampling, delayed strobe signal would affect the accuracy of bit stripping/stuffing
      | 2. The BER performance degrades significantly even with frame size 2 and 4
  note: Baseband implementation of the Symbol Timing Synchronization listed in Chapter 8.4
      | of "Digital Communications- A Discrete-Time Approach" by Michael Rice. See Appendix
      | C.2 of the same book for the details of PLL design.
  note: To determine phase error detector gain K_p, See Equation 8.42 &
      | Figure 8.4.7 of "Digital Communications - A Discrete-Time Approach"
      | by Michael Rice.
  DataIn : Inport
  Integer Delay1 : Delay  DelayLength=1
  Integer Delay2 : Delay  DelayLength=1
  Interpolation Filter : MATLAB Function  TreatAsAtomicUnit=on
  Loop Filter : Subsystem  mask{BnTs=0.01, zeta=1, Kp=sdrqpskrx.TimingRecTEDGain, K0=sdrqpskrx.TimingRecCompensateGain, N=sdrqpskrx.Upsampling/sdrqpskrx.Downsampling}
      mask prompts: BnTs "Loop Bandwidth"; zeta "Loop Damping Factor"; Kp "Phase Detector Gain (Kp)"; K0 "DDS gain (K0)"; N "Number of Samples/symbol (N)"
      mask init:
      | % See C.57 to C.61 in Michael Rice's "Digital Communications 
      | % - A Discrete-Time Approach" for details
      | theta = BnTs/(zeta+0.25/zeta)/N;
      | d = 1 + 2*zeta*theta + theta*theta;
      | K1 = 4*zeta*theta/d;
      | K2 = 4*theta*theta/d;
      | K1 = K1/(Kp*K0);
      | K2 = K2/(Kp*K0);
      mask Display: disp('Loop Filter');
  NCO Control : MATLAB Function
  Timing Error Detector : MATLAB Function  TreatAsAtomicUnit=on
  DataOut : Outport
  ClkOut : Outport  Port=2
  wires:
  DataIn/1 -> Interpolation Filter/1(In)
  NCO Control/2(mu) -> Integer Delay2/1
  Integer Delay1/1 -> ClkOut/1, Timing Error Detector/2(strobe)
  NCO Control/1(Underflow) -> Integer Delay1/1
  Interpolation Filter/1(Out) -> DataOut/1, Timing Error Detector/1(In)
  Loop Filter/1(v) -> NCO Control/1(Delta)
  Timing Error Detector/1(e) -> Loop Filter/1(e)
  Integer Delay2/1 -> Interpolation Filter/2(mu)

== system QPSK_ad9361_Solution/QPSK TX/Bit Generation/Barker Code SS ==
  Constant Barker Code : Constant  Value=|  VectorParams1D=off
      | [+1 +1 +1 +1 +1 -1 -1 +1 +1 -1 +1 -1 +1
      | ].' > 0  % Bipolar to Unipolar Conversion
      settings: SamplingMode=Frame based
  Data Type Conversion : DataTypeConversion  OutDataTypeStr=double
  Out : Outport
  wires:
  Data Type Conversion/1 -> Out/1
  Constant Barker Code/1 -> Data Type Conversion/1

== system QPSK_ad9361_Solution/QPSK TX/Bit Generation/Message Source ==
  Bernoulli Binary Generator : commrandsrc2/Bernoulli Binary Generator  P=0.5  seed=61  Ts=sdrqpsktx.FrameTime/(sdrqpsktx.DataLength-sdrqpsktx.MsgLength)  frameBased=on  sampPerFrame=sdrqpsktx.DataLength-sdrqpsktx.MsgLength  orient=off  outDataType=double
      settings: SourceProductName=Communications Toolbox  SourceProductBaseCode=CM
  Matrix Concatenate : Concatenate  Mode=Multidimensional array
  Message Generator : MATLAB Function  TreatAsAtomicUnit=on
  Out : Outport
  wires:
  Matrix Concatenate/1 -> Out/1
  Bernoulli Binary Generator/1 -> Matrix Concatenate/2
  Message Generator/1(msg) -> Matrix Concatenate/1

== system QPSK_ad9361_Solution/ADI9361_rx1/ADC_RX/ADC_I/Quantizer1 ==
  u : Inport
  Abs : Abs
  Idealized ADC quantizer : simulink_extras/Additional Discrete/Idealized ADC quantizer  NumberOfConverterBits=3  Vmin=0  Vmax=.8  OutputDataType=double  OutputNegativeValues=off
      settings: SourceProductName=Simulink
  Product : Product
  Saturation : Saturate  UpperLimit=0.41
  Sign : Signum
  y : Outport
  wires:
  u/1 -> Sign/1, Abs/1
  Saturation/1 -> Idealized ADC quantizer/1
  Idealized ADC quantizer/1 -> Product/1
  Sign/1 -> Product/2
  Abs/1 -> Saturation/1
  Product/1 -> y/1

== system QPSK_ad9361_Solution/ADI9361_rx1/ADC_RX/ADC_Q/Quantizer1 ==
  u : Inport
  Abs : Abs
  Idealized ADC quantizer : simulink_extras/Additional Discrete/Idealized ADC quantizer  NumberOfConverterBits=3  Vmin=0  Vmax=.8  OutputDataType=double  OutputNegativeValues=off
      settings: SourceProductName=Simulink
  Product : Product
  Saturation : Saturate  UpperLimit=0.41
  Sign : Signum
  y : Outport
  wires:
  u/1 -> Sign/1, Abs/1
  Saturation/1 -> Idealized ADC quantizer/1
  Idealized ADC quantizer/1 -> Product/1
  Sign/1 -> Product/2
  Abs/1 -> Saturation/1
  Product/1 -> y/1

== system QPSK_ad9361_Solution/ADI9361_rx1/DDC_Filters_RX/Hm1/Hm1 ==
  In : Inport
  Hm1 : dspmlti4/FIR Decimation  FilterSource=Filter object  h=fir1(35,0.4)  D=2  filtStruct=Direct form  FilterObject=ad9361_rx_pars.Hm1_rx  framing=Allow multirate processing  inputOffset=0  outputBufInitCond=0  roundingMode=Floor  overflowMode=off  firstCoeffDataTypeStr=Inherit: Same word length as input  firstCoeffMin=[]  firstCoeffMax=[]  firstCoeffLastDataTypeStr=Inherit: Same word length as input  outputDataTypeStr=Inherit: Same as accumulator  outputMin=[]  outputMax=[]  outputLastDataTypeStr=Inherit: Same as accumulator
  Out : Outport
  wires:
  In/1 -> Hm1/1
  Hm1/1 -> Out/1

== system QPSK_ad9361_Solution/ADI9361_rx1/DDC_Filters_RX/Hm1/NoFilter ==
  In : Inport
  Out : Outport
  wires:
  In/1 -> Out/1

== system QPSK_ad9361_Solution/ADI9361_rx1/DDC_Filters_RX/Hm2/Hm2 ==
  In : Inport
  Data Type Conversion3 : DataTypeConversion  OutDataTypeStr=fixdt(1,16,14)  RndMeth=Round
  Hm2 : dspmlti4/FIR Decimation  FilterSource=Filter object  h=fir1(35,0.4)  D=2  filtStruct=Direct form  FilterObject=ad9361_rx_pars.Hm2_rx  framing=Allow multirate processing  inputOffset=0  outputBufInitCond=0  roundingMode=Floor  overflowMode=off  firstCoeffDataTypeStr=Inherit: Same word length as input  firstCoeffMin=[]  firstCoeffMax=[]  firstCoeffLastDataTypeStr=Inherit: Same word length as input  outputDataTypeStr=Inherit: Same as accumulator  outputMin=[]  outputMax=[]  outputLastDataTypeStr=Inherit: Same as accumulator
  Out : Outport
  wires:
  In/1 -> Data Type Conversion3/1
  Hm2/1 -> Out/1
  Data Type Conversion3/1 -> Hm2/1

== system QPSK_ad9361_Solution/ADI9361_rx1/DDC_Filters_RX/Hm2/NoFilter ==
  In : Inport
  Data Type Conversion3 : DataTypeConversion  OutDataTypeStr=fixdt(1,16,14)  RndMeth=Round
  Out : Outport
  wires:
  In/1 -> Data Type Conversion3/1
  Data Type Conversion3/1 -> Out/1

== system QPSK_ad9361_Solution/ADI9361_rx1/DDC_Filters_RX/Hm3/Hm3 ==
  In : Inport
  Mh3 : dspmlti4/FIR Decimation  FilterSource=Filter object  h=fir1(35,0.4)  D=2  filtStruct=Direct form  FilterObject=ad9361_rx_pars.Hm3_rx  framing=Allow multirate processing  inputOffset=0  outputBufInitCond=0  roundingMode=Floor  overflowMode=off  firstCoeffDataTypeStr=Inherit: Same word length as input  firstCoeffMin=[]  firstCoeffMax=[]  firstCoeffLastDataTypeStr=Inherit: Same word length as input  outputDataTypeStr=Inherit: Same as accumulator  outputMin=[]  outputMax=[]  outputLastDataTypeStr=Inherit: Same as accumulator
  Out : Outport
  wires:
  In/1 -> Mh3/1
  Mh3/1 -> Out/1

== system QPSK_ad9361_Solution/ADI9361_rx1/DDC_Filters_RX/Hm3/NoFilter ==
  In : Inport
  Out : Outport
  wires:
  In/1 -> Out/1

== system QPSK_ad9361_Solution/ADI9361_rx1/DDC_Filters_RX/Hm4/Hm4 ==
  In1 : Inport
  Data Type Conversion : DataTypeConversion  OutDataTypeStr=fixdt(1,4,2)  RndMeth=Round
  Hm1 : dspmlti4/FIR Decimation  FilterSource=Filter object  h=fir1(35,0.4)  D=2  filtStruct=Direct form  FilterObject=ad9361_rx_pars.Hm4_rx  framing=Allow multirate processing  inputOffset=0  outputBufInitCond=0  roundingMode=Floor  overflowMode=off  firstCoeffDataTypeStr=Inherit: Same word length as input  firstCoeffMin=[]  firstCoeffMax=[]  firstCoeffLastDataTypeStr=Inherit: Same word length as input  outputDataTypeStr=Inherit: Same as accumulator  outputMin=[]  outputMax=[]  outputLastDataTypeStr=Inherit: Same as accumulator
  Out1 : Outport
  wires:
  In1/1 -> Data Type Conversion/1
  Hm1/1 -> Out1/1
  Data Type Conversion/1 -> Hm1/1

== system QPSK_ad9361_Solution/ADI9361_rx1/DDC_Filters_RX/Hm4/NoFilter ==
  In1 : Inport
  Data Type Conversion : DataTypeConversion  OutDataTypeStr=fixdt(1,4,2)  RndMeth=Round
  Out1 : Outport
  wires:
  In1/1 -> Data Type Conversion/1
  Data Type Conversion/1 -> Out1/1

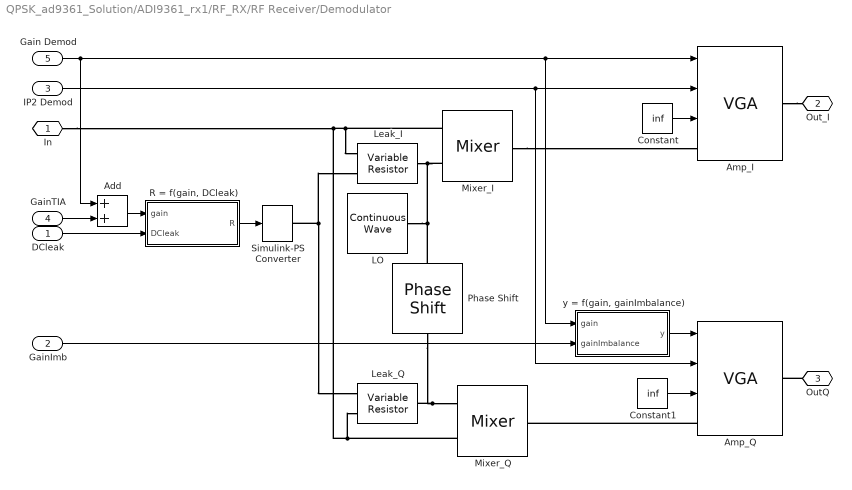
== system QPSK_ad9361_Solution/ADI9361_rx1/RF_RX/RF Receiver/Demodulator ==
  DCleak : Inport
  GainImb : Inport  Port=2
  IP2 Demod : Inport  Port=3
  GainTIA : Inport  Port=4
  Gain Demod : Inport  Port=5
  Add : Sum
  Amp_I : simrfV2elements/VGA  classname=vga  Zin=100  Zout=100  IO=Input  InternalGrounding=on
      settings: SourceProductName=RF Blockset  SourceProductBaseCode=RB
  Amp_Q : simrfV2elements/VGA  classname=vga  Zin=100  Zout=100  IO=Input  InternalGrounding=on
      settings: SourceProductName=RF Blockset  SourceProductBaseCode=RB
  Constant : Constant  Value=inf
  Constant1 : Constant  Value=inf
  LO : simrfV2sources1/Continuous Wave  CWSourceType=Ideal voltage  Z0=0  IVoltage=1/sqrt(2) V  ICurrent=0 A  MagPower=1 W  QVoltage=0 V  QCurrent=0 A  AnglePower=0  CarrierFreq=RF Hz  InternalGrounding=on
      settings: SourceProductName=RF Blockset  SourceProductBaseCode=RB
  Leak_I : fl_lib/Electrical/Electrical Elements/Variable Resistor  Rmin=0 Ohm  i_specify=off  i_priority=High  i=0 A  v_specify=off  v_priority=High  v=0 V
  Leak_Q : fl_lib/Electrical/Electrical Elements/Variable Resistor  Rmin=0 Ohm  i_specify=off  i_priority=High  i=0 A  v_specify=off  v_priority=High  v=0 V
  Mixer_I : simrfV2elements/Mixer  classname=mixer  Source_linear_gain=Available power gain  linear_gain=0 dB  Zin=100  Zout=100  ZLO=inf  Source_Poly=Even and odd order  Poly_Coeffs=[0 1]  IPType=Output  IP2=Inf dBm  IP3=Inf dBm  P1dB=Inf dBm  Psat=Inf dBm  Gcomp=Inf dBm  NF=0  InternalGrounding=on
      settings: SourceProductName=RF Blockset  SourceProductBaseCode=RB
  Mixer_Q : simrfV2elements/Mixer  classname=mixer  Source_linear_gain=Available power gain  linear_gain=0 dB  Zin=100  Zout=100  ZLO=inf  Source_Poly=Even and odd order  Poly_Coeffs=[0 1]  IPType=Output  IP2=Inf dBm  IP3=Inf dBm  P1dB=Inf dBm  Psat=Inf dBm  Gcomp=Inf dBm  NF=0  InternalGrounding=on
      settings: SourceProductName=RF Blockset  SourceProductBaseCode=RB
  Phase Shift : simrfV2elements/Phase Shift  PhaseShift=90 deg  InternalGrounding=on
      settings: SourceProductName=RF Blockset  SourceProductBaseCode=RB
  "R = f(gain, DCleak)" : Subsystem
  Simulink-PS Converter : nesl_utility/Simulink-PS Converter  PhysicalDomain=network_engine_domain  SubClassName=ps_input  LeftPortType=input  RightPortType=output  PseudoPeriodic=off  Frequencies=[]  NoiseDistribution=none  NoiseParameters=[]  Unit=1  AffineConversion=off  InputFiltering=off  SimscapeFilterOrder=1  InputFilterTimeConstant=0.001  UdotUserProvided=1
  "y = f(gain, gainImbalance)" : Subsystem
  In : PMIOPort  Side=Left
  Out_I : PMIOPort  Port=2  Side=Right
  OutQ : PMIOPort  Port=3  Side=Right
  wires:
  Gain Demod/1 -> "y = f(gain, gainImbalance)"/1(gain), Amp_I/1, Add/1
  IP2 Demod/1 -> Amp_Q/2, Amp_I/2
  "R = f(gain, DCleak)"/1(R) -> Simulink-PS Converter/1
  GainTIA/1 -> Add/2
  Add/1 -> "R = f(gain, DCleak)"/1(gain)
  GainImb/1 -> "y = f(gain, gainImbalance)"/2(gainImbalance)
  DCleak/1 -> "R = f(gain, DCleak)"/2(DCleak)
  "y = f(gain, gainImbalance)"/1(y) -> Amp_Q/1
  Constant/1 -> Amp_I/3
  Constant1/1 -> Amp_Q/3
  connections:
  Phase Shift/RConn1 -- Mixer_Q/LConn2 -- Leak_Q/RConn1
  Mixer_I/LConn2 -- Leak_I/RConn1 -- LO/LConn1 -- Phase Shift/LConn1
  Mixer_Q/LConn1 -- Leak_Q/LConn2 -- In/RConn1 -- Leak_I/LConn2 -- Mixer_I/LConn1
  Amp_I/RConn1 -- Out_I/RConn1
  OutQ/RConn1 -- Amp_Q/RConn1
  Mixer_I/RConn1 -- Amp_I/LConn1
  Amp_Q/LConn1 -- Mixer_Q/RConn1
  Simulink-PS Converter/RConn1 -- Leak_Q/LConn1 -- Leak_I/LConn1

== system QPSK_ad9361_Solution/ADI9361_rx1/RF_RX/RF Receiver/External LNA ==
  ExternalLNA on/off : Inport
  Bypass : simrfV2junction1/Switch  classname=switch  Ron=0 Ohm  Roff=inf Ohm  Vthres=0.5 V
      settings: SourceProductName=RF Blockset  SourceProductBaseCode=RB
  Invert Control : Subsystem
  LNA : simrfV2elements/Amplifier  classname=amplifier  DataSource=Data file  File=simrfV2_unitygain.s2p  Paramtype=S-parameters  Sparam=[0 0;1 0]  SparamFreq=1e9 Hz  SparamZ0=50  Residues=0  Poles=0  DF={0 0; 1 0}  Source_linear_gain=Available power gain  linear_gain=10 dB  Zin=50  Zout=50  Source_Poly=Even and odd order  Poly_Coeffs=[0 1]  IPType=Output  IP2=inf dBm  IP3=inf dBm  P1dB=inf dBm  Psat=inf dBm  Gcomp=inf dBm  NF=0  InternalGrounding=on  SourceFreq=Extracted from data source  PlotFreq=[1e9:1e6:3e9] Hz  PlotType=X-Y plane  YParam1=S11  YFormat1=Magnitude (decibels)  YParam2=None  YFormat2=Magnitude (decibels)  YOption=Linear  XOption=Linear  SparamRepresentation=Time domain (rationalfit)  FitTol=-40  FitOpt=Fit individually  AutoImpulseLength=off  ImpulseLength=0 s
      settings: SourceProductName=RF Blockset  SourceProductBaseCode=RB
  LNA on input : simrfV2junction1/Switch  classname=switch  Ron=0 Ohm  Roff=inf Ohm  Vthres=0.5 V
      settings: SourceProductName=RF Blockset  SourceProductBaseCode=RB
  LNA on ouput : simrfV2junction1/Switch  classname=switch  Ron=0 Ohm  Roff=inf Ohm  Vthres=0.5 V
      settings: SourceProductName=RF Blockset  SourceProductBaseCode=RB
  in : PMIOPort  Side=Left
  out : PMIOPort  Port=2  Side=Right
  wires:
  ExternalLNA on/off/1 -> LNA on ouput/1, LNA on input/1, Invert Control/1(In)
  Invert Control/1(Out) -> Bypass/1
  connections:
  Bypass/RConn1 -- out/RConn1 -- LNA on ouput/RConn1
  LNA on input/LConn1 -- Bypass/LConn1 -- in/RConn1
  LNA on input/RConn1 -- LNA/LConn1
  LNA/RConn1 -- LNA on ouput/LConn1

== system QPSK_ad9361_Solution/ADI9361_rx1/RF_RX/RF Receiver/RF Non Idealities ==
  LPF : Inport
  TIA : Inport  Port=2
  Demod : Inport  Port=3
  LNA : Inport  Port=4
  DetectChange : Subsystem
  RF Non Idealities : Subsystem
  DCLeakage : Outport
  GainImbalance : Outport  Port=2
  IP2 : Outport  Port=3
  IP3 : Outport  Port=4
  wires:
  TIA/1 -> RF Non Idealities/3(TIA), DetectChange/3(In3)
  LPF/1 -> RF Non Idealities/4(LPF), DetectChange/4(In4)
  Demod/1 -> RF Non Idealities/2(Demod), DetectChange/2(In2)
  LNA/1 -> RF Non Idealities/1(LNA), DetectChange/1(In1)
  RF Non Idealities/1(DCLeakage) -> DCLeakage/1
  RF Non Idealities/2(GainImbalance) -> GainImbalance/1
  RF Non Idealities/3(IP2) -> IP2/1
  RF Non Idealities/4(IP3) -> IP3/1
  DetectChange/1(Trigger) -> RF Non Idealities/Trigger

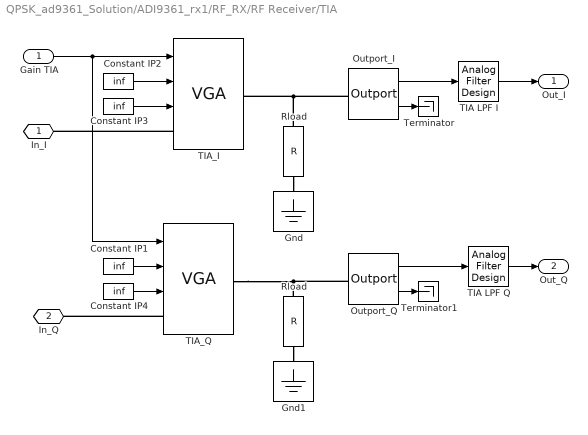
== system QPSK_ad9361_Solution/ADI9361_rx1/RF_RX/RF Receiver/TIA ==
  Gain TIA : Inport
  " Rload" : simrfV2elements/R  classname=resistor  Resistance=100 Ohm  AddNoise=on
      settings: SourceProductName=RF Blockset  SourceProductBaseCode=RB
  Constant IP{1..4} (4 alike) : Constant  Value=inf
  Gnd : fl_lib/Electrical/Electrical Elements/Electrical Reference
  Gnd1 : fl_lib/Electrical/Electrical Elements/Electrical Reference
  Outport_I : simrfV2util1/Outport  SensorType=Ideal voltage  OutputFormat=In-phase and Quadrature Baseband  CarrierFreq=0 Hz  ZL=Inf  InternalGrounding=on  StepSize=-1 s  AutoStep=off
      settings: SourceProductName=RF Blockset  SourceProductBaseCode=RB
  Outport_Q : simrfV2util1/Outport  SensorType=Ideal voltage  OutputFormat=In-phase and Quadrature Baseband  CarrierFreq=0 Hz  ZL=Inf  InternalGrounding=on  StepSize=-1 s  AutoStep=off
      settings: SourceProductName=RF Blockset  SourceProductBaseCode=RB
  Rload : simrfV2elements/R  classname=resistor  Resistance=100 Ohm  AddNoise=on
      settings: SourceProductName=RF Blockset  SourceProductBaseCode=RB
  TIA LPF I : dsparch4/Analog Filter Design  method=Butterworth  filttype=Lowpass  N=1  Wlo=2.5*ad9361_rx_pars.Fpass*2*pi  Whi=80  Rp=2  Rs=40
  TIA LPF Q : dsparch4/Analog Filter Design  method=Butterworth  filttype=Lowpass  N=1  Wlo=2.5*ad9361_rx_pars.Fpass*2*pi  Whi=80  Rp=2  Rs=40
  TIA_I : simrfV2elements/VGA  classname=vga  Zin=100  Zout=100  IO=Input  InternalGrounding=on
      settings: SourceProductName=RF Blockset  SourceProductBaseCode=RB
  TIA_Q : simrfV2elements/VGA  classname=vga  Zin=100  Zout=100  IO=Input  InternalGrounding=on
      settings: SourceProductName=RF Blockset  SourceProductBaseCode=RB
  Terminator : Terminator
  Terminator1 : Terminator
  In_I : PMIOPort  Side=Left
  In_Q : PMIOPort  Port=2  Side=Left
  Out_I : Outport
  Out_Q : Outport  Port=2
  wires:
  Outport_Q/1 -> TIA LPF Q/1
  Outport_I/1 -> TIA LPF I/1
  Outport_I/2 -> Terminator/1
  Outport_Q/2 -> Terminator1/1
  Gain TIA/1 -> TIA_Q/1, TIA_I/1
  TIA LPF I/1 -> Out_I/1
  TIA LPF Q/1 -> Out_Q/1
  Constant IP2/1 -> TIA_I/2
  Constant IP3/1 -> TIA_I/3
  Constant IP1/1 -> TIA_Q/2
  Constant IP4/1 -> TIA_Q/3
  connections:
  TIA_I/LConn1 -- In_I/RConn1
  TIA_Q/LConn1 -- In_Q/RConn1
  Outport_I/LConn1 -- Rload/LConn1 -- TIA_I/RConn1
  Outport_Q/LConn1 -- TIA_Q/RConn1 -- " Rload"/LConn1
  Rload/RConn1 -- Gnd/LConn1
  " Rload"/RConn1 -- Gnd1/LConn1

== system QPSK_ad9361_Solution/ADI9361_tx1/DUC_Filters_TX/Hm1/Hm1 ==
  In : Inport
  Hm1 : dspmlti4/FIR Interpolation  FilterSource=Filter object  h=fir1(15,1/4)  L=3  FilterObject=ad9361_tx_pars.Hm1_tx  framing=Allow multirate processing  outputBufInitCond=0  roundingMode=Floor  overflowMode=off  firstCoeffDataTypeStr=Inherit: Same word length as input  firstCoeffMin=[]  firstCoeffMax=[]  firstCoeffLastDataTypeStr=Inherit: Same word length as input  outputDataTypeStr=Inherit: Same as accumulator  outputMin=[]  outputMax=[]  outputLastDataTypeStr=Inherit: Same as accumulator
      settings: SourceProductName=DSP System Toolbox
  Out : Outport
  wires:
  Hm1/1 -> Out/1
  In/1 -> Hm1/1

== system QPSK_ad9361_Solution/ADI9361_tx1/DUC_Filters_TX/Hm1/NoFilter ==
  In : Inport
  Out : Outport
  wires:
  In/1 -> Out/1

== system QPSK_ad9361_Solution/ADI9361_tx1/DUC_Filters_TX/Hm2/Hm2 ==
  In : Inport
  Hm2 : dspmlti4/FIR Interpolation  FilterSource=Filter object  h=fir1(15,1/4)  L=3  FilterObject=ad9361_tx_pars.Hm2_tx  framing=Allow multirate processing  outputBufInitCond=0  roundingMode=Floor  overflowMode=off  firstCoeffDataTypeStr=Inherit: Same word length as input  firstCoeffMin=[]  firstCoeffMax=[]  firstCoeffLastDataTypeStr=Inherit: Same word length as input  outputDataTypeStr=Inherit: Same as accumulator  outputMin=[]  outputMax=[]  outputLastDataTypeStr=Inherit: Same as accumulator
      settings: SourceProductName=DSP System Toolbox
  Out : Outport
  wires:
  Hm2/1 -> Out/1
  In/1 -> Hm2/1

== system QPSK_ad9361_Solution/ADI9361_tx1/DUC_Filters_TX/Hm2/NoFilter ==
  In : Inport
  Out : Outport
  wires:
  In/1 -> Out/1
